simulink model "Final_Real_Model_Position_plus_PID"  (R2024a)
settings: Solver=FixedStepAuto  StartTime=0.0  StopTime=inf  FixedStep=0.005  RelTol=1e-3  EnableMultiTasking=on
libraries: arduinolib x5, arduinosensorlib x1
settings Model: NumberOfSteps=2  ExtModeTrigDuration=2  Creator=Taha  LastModifiedBy=mahmoud eldawakhly
settings OptimizationCC: EnhancedBackFolding=on  PassReuseOutputArgsThreshold=0  MaxStackSize=64  OptimizeBlockOrder=speed  DifferentSizesBufferReuse=on  OptimizationCustomize=off
settings DebuggingCC: ParameterPrecisionLossMsg=none  ParameterTunabilityLossMsg=error
settings HardwareCC: ProdBitPerInt=16  ProdBitPerPointer=16  ProdBitPerSizeT=16  ProdBitPerPtrDiffT=16  ProdLargestAtomicFloat=None  ProdWordSize=8  ProdHWDeviceType=Atmel->AVR  UseEmbeddedCoderFeatures=off  UseSimulinkCoderFeatures=off
settings SFSimCC: MATLABDynamicMemAlloc=off
settings RTWCC: Description=Embedded Coder  SystemTargetFile=ert.tlc  HardwareBoard=Arduino Uno  TemplateMakefile=ert_default_tmf  RTWVerbose=off  Toolchain=Arduino AVR  BuildConfiguration=Faster Runs  GPUComputeCapability=3.5
settings CodeAppCC: ForceParamTrailComments=on  OperatorAnnotations=on
settings ERTTargetCC: ERTCustomFileBanners=off  SupportContinuousTime=on  SupportNonInlinedSFcns=on  RemoveResetFunc=off  SupportVariableSizeSignals=on  ModelStepFunctionPrototypeControlCompliant=off  ExtModeTransport=3  ExtModeStaticAlloc=on  ExtModeAutomaticAllocSize=off  ExtModeStaticAllocSize=250  ExtModeMexFile=ext_xcp  ExtModeIntrfLevel=Level2 - Open  ERTSrcFileBannerTemplate=codertarget_code_template.cgt  ERTHdrFileBannerTemplate=codertarget_code_template.cgt  ERTDataSrcFileTemplate=codertarget_code_template.cgt  ERTDataHdrFileTemplate=codertarget_code_template.cgt

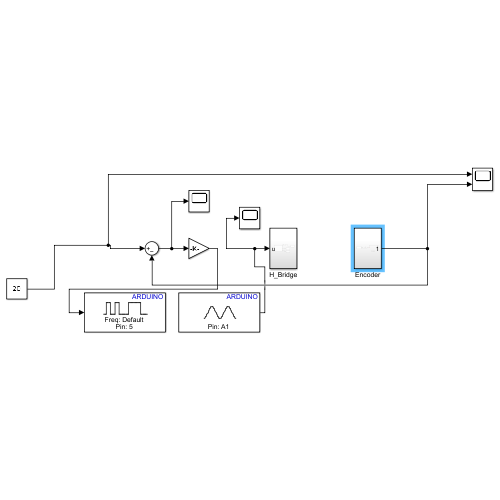
[thumbnail: Simulink's stored preview of the top-level diagram]
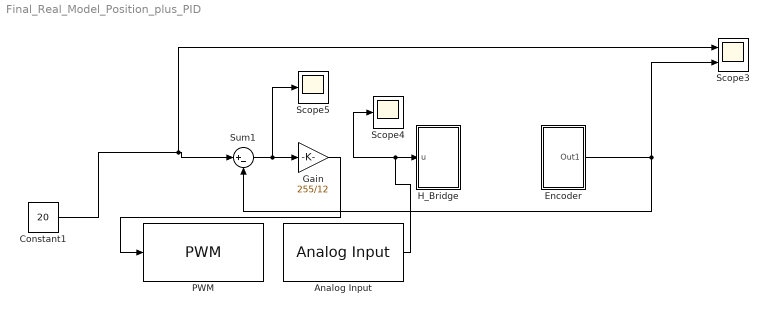
== system Final_Real_Model_Position_plus_PID ==
  Analog Input : arduinolib/Analog Input  pinNumber=1  ReadResultsOnly=off  ConversionTriggerSource=Software  ExternalTriggerType=uint32( 0 )  OutputDataType=uint16  EnableConversionCompleteNotify=off  EnableOuputStatus=off  SampleTime=-1  blockPlatform=arduino
  Constant1 : Constant  Value=20
  Encoder : Subsystem
  Gain : Gain  Gain=255/12
  H_Bridge : Subsystem
  PWM : arduinolib/PWM  pinNumber=5  frequencyType=Default  desiredFrequency=490.2  achievableFrequency=490.2
  Scope3 : Scope  NumInputPorts=2
  Scope4 : Scope
  Scope5 : Scope
  Sum1 : Sum  Inputs=|+-
  wires:
  Encoder/1(Out1) -> Scope3/2, Sum1/2
  Sum1/1 -> Gain/1, Scope5/1
  Analog Input/1 -> Scope4/1, H_Bridge/1(u)
  Constant1/1 -> Scope3/1, Sum1/1
  Gain/1 -> PWM/1

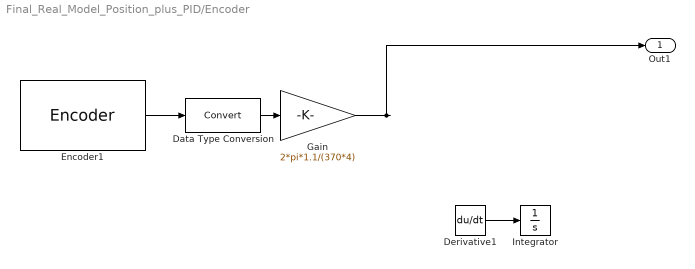
== system Final_Real_Model_Position_plus_PID/Encoder ==
  Data Type Conversion : DataTypeConversion  SaturateOnIntegerOverflow=off  RndMeth=Floor
  Derivative1 : Derivative
  Encoder1 : arduinosensorlib/Encoder  InputA=2  InputB=3  Mode=No reset  SampleTime=-1
  Gain : Gain  Gain=2*pi*1.1/(370*4)  OutDataTypeStr=double
  Integrator : Integrator
  Out1 : Outport
  wires:
  Data Type Conversion/1 -> Gain/1
  Encoder1/1 -> Data Type Conversion/1
  Gain/1 -> Out1/1
  Derivative1/1 -> Integrator/1

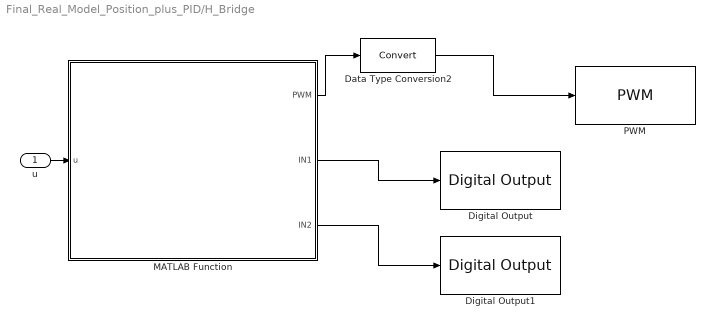
== system Final_Real_Model_Position_plus_PID/H_Bridge ==
  u : Inport
  Data Type Conversion2 : DataTypeConversion  SaturateOnIntegerOverflow=off  RndMeth=Floor
  Digital Output : arduinolib/Digital Output  pinNumber=11  Direction=output  blockPlatform=arduino
  Digital Output1 : arduinolib/Digital Output  pinNumber=10  Direction=output  blockPlatform=arduino
  MATLAB Function : MATLAB Function  TreatAsAtomicUnit=on
  PWM : arduinolib/PWM  pinNumber=9  frequencyType=Specify  desiredFrequency=2000  achievableFrequency=2000
  wires:
  MATLAB Function/1(PWM) -> Data Type Conversion2/1
  MATLAB Function/3(IN2) -> Digital Output1/1
  u/1 -> MATLAB Function/1(u)
  MATLAB Function/2(IN1) -> Digital Output/1
  Data Type Conversion2/1 -> PWM/1

== matlab function Final_Real_Model_Position_plus_PID/H_Bridge/MATLAB Function ==
  data: u input; PWM output; IN1 output; IN2 output
function [PWM,IN1,IN2]=fcn1(u)
PWM= abs(u);
if u<0
IN1=1; IN2=0;
elseif u>0
IN1=0; IN2=1;
else
IN1=0; IN2=0;
end
